simulink model "SC228_TrackedASModelUnitTest"  (R2018b)
settings: Solver=VariableStepAuto  StartTime=0.0  StopTime=10.0  RelTol=1e-3
undefined symbols (not defined in the file or in its folder): ac1dyn_alt0_ft, ac1dyn_con, ac1dyn_lat0_rad, ac1dyn_lon0_rad, ac2dyn_alt0_ft, ac2dyn_con, ac2dyn_lat0_rad, ac2dyn_lon0_rad, ddh_ftps2, dh_ftps, dv_ftps2, e_ft, Edot_ftps, h_ft, hdot_ftps, latLonAltState, n_ft, Ndot_ftps, p_radps, phi_rad, phidot_radps, psi_rad, psidot_radps, q_radps, r_radps, theta_rad, thetadot_radps, uas_tcas_trckd_altQuant_ft, uas_tcas_trckd_bearing_Breakpoints_deg, uas_tcas_trckd_bearing_Max_deg, uas_tcas_trckd_bearing_Sigma_deg, uas_tcas_trckd_dt_s, uas_tcas_trckd_FOR_elev_max_deg, uas_tcas_trckd_FOR_elev_min_deg, uas_tcas_trckd_probDetect, uas_tcas_trckd_psi_bias_ft, uas_tcas_trckd_psi_stddev_ft, uas_tcas_trckd_psidot_bias_radps, uas_tcas_trckd_psidot_stddev_ftps, uas_tcas_trckd_randProbSeed, uas_tcas_trckd_reported_errorCovRBA, uas_tcas_trckd_rng_bias_ft, uas_tcas_trckd_rng_random_stddev_ft, uas_tcas_trckd_seed1, uas_tcas_trckd_seed2, uas_tcas_trckd_seed3, uas_tcas_trckd_seed4, uas_tcas_trckd_sns_max_front_range_ft, uas_tcas_trckd_sns_max_range_ft, uas_tcas_trckd_sns_max_rear_range_ft, uas_tcas_trckd_sns_max_side_range_ft, uas_tcas_trckd_tauThreshold_sec, uas_tcas_trckd_updateRate_sec, v_ftps, vdot_fpss
libraries: simulink x20, dspmtrx3 x1
(part 1 of 2)
settings Model: Creator=PE29732  LastModifiedBy=PE29732

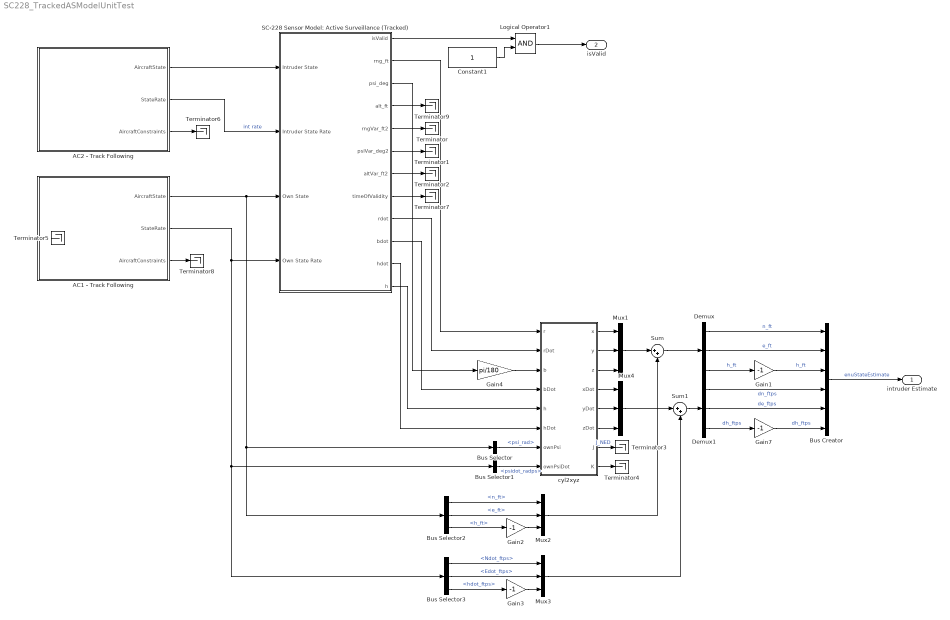
== system SC228_TrackedASModelUnitTest ==
  AC1 - Track Following : Subsystem  mask(Basic Aircraft Dynamic Model){ts_dynamics=0.1, lat0_rad=ac1dyn_lat0_rad, lon0_rad=ac1dyn_lon0_rad, alt_ft=ac1dyn_alt0_ft, v_ftps_max=ac1dyn_con.maxAirspeed_ftps, v_ftps_min=ac1dyn_con.minAirspeed_ftps, dv_ftpss_max=ac1dyn_con.maxAcceleration_ftpss, dv_ftpss_min=ac1dyn_con.minAcceleration_ftpss, dh_ftps_max=ac1dyn_con.maxVerticalRate_ftps, dh_ftps_min=ac1dyn_con.minVerticalRate_ftps, q_radps_max=ac1dyn_con.maxPitchRate_radps, phi_rad_max=ac1dyn_con.maxBankAngle_rad, dphi_radps_max=ac1dyn_con.maxRollRate_radps, r_radps_max=ac1dyn_con.maxYawRate_radps, pNUM=ac1dyn_con.dynamicsNumeratorRollRate, pDEN=ac1dyn_con.dynamicsDenominatorRollRate, hNUM=ac1dyn_con.dynamicsNumeratorVerticalRate, hDEN=ac1dyn_con.dynamicsDenominatorVerticalRate, rNUM=ac1dyn_con.dynamicsNumeratorYawRate, rDEN=ac1dyn_con.dynamicsDenominatorYawRate}
      mask prompts: ts_dynamics "Dynamics update parameter"; lat0_rad "Latitude of ENU origin (rad)"; lon0_rad "Longitude of ENU origin (rad)"; alt_ft "Height of ENU origin (ft)"; v_ftps_max "Maximum airspeed (ft/s)"; v_ftps_min "Minimum airspeed (ft/s)"; dv_ftpss_max "Maximum acceleration (ft/s/s)"; dv_ftpss_min "Miniimum acceleration (ft/s/s)"; dh_ftps_max "Maximum vertical rate (ft/s)"; dh_ftps_min "Minimum vertical rate (ft/s)"; q_radps_max "Maximum pitch rate (rad/s)"; phi_rad_max "Maximum bank angle (rad)"; dphi_radps_max "Maximum roll rate (rad/s)"; r_radps_max "Maximum yaw rate (rad/s)"; pNUM "Roll rate discrete dynamics numerator (2x1)"; pDEN "Roll rate discrete dynamics denominator (1x1)"; hNUM "Vertical rate discrete dynamics numerator (2x1)"; hDEN "Vertical rate discrete dynamics denominator (1x1)"; rNUM "Yaw rate discrete dynamics numerator (2x1)"; rDEN "Yaw rate discrete dynamics denominator (1x1)"
      mask help:
      | Propagates the aircraft dynamics using 6DOF equations of motion.
      |
      | The class Simple6DOF can be used to programmatically set the parameters of Basic Aircraft Dynamcis blocks.
      mask Help:
      | Propagates the aircraft dynamics using 6DOF equations of motion.
      | 
      | The class Simple6DOF can be used to programmatically set the parameters of Basic Aircraft Dynamcis blocks.
      mask DialogControl ParameterTabVar0 Prompt: Main
      mask DialogControl ParameterTabVar01 Prompt: Constraints
  AC2 - Track Following : Subsystem  mask(Basic Aircraft Dynamic Model){ts_dynamics=0.1, lat0_rad=ac2dyn_lat0_rad, lon0_rad=ac2dyn_lon0_rad, alt_ft=ac2dyn_alt0_ft, v_ftps_max=ac2dyn_con.maxAirspeed_ftps, v_ftps_min=ac2dyn_con.minAirspeed_ftps, dv_ftpss_max=ac2dyn_con.maxAcceleration_ftpss, dv_ftpss_min=ac2dyn_con.minAcceleration_ftpss, dh_ftps_max=ac2dyn_con.maxVerticalRate_ftps, dh_ftps_min=ac2dyn_con.minVerticalRate_ftps, q_radps_max=ac2dyn_con.maxPitchRate_radps, phi_rad_max=ac2dyn_con.maxBankAngle_rad, dphi_radps_max=ac2dyn_con.maxRollRate_radps, r_radps_max=ac2dyn_con.maxYawRate_radps, pNUM=ac2dyn_con.dynamicsNumeratorRollRate, pDEN=ac2dyn_con.dynamicsDenominatorRollRate, hNUM=ac2dyn_con.dynamicsNumeratorVerticalRate, hDEN=ac2dyn_con.dynamicsDenominatorVerticalRate, rNUM=ac2dyn_con.dynamicsNumeratorYawRate, rDEN=ac2dyn_con.dynamicsDenominatorYawRate}
      mask prompts: ts_dynamics "Dynamics update parameter"; lat0_rad "Latitude of ENU origin (rad)"; lon0_rad "Longitude of ENU origin (rad)"; alt_ft "Height of ENU origin (ft)"; v_ftps_max "Maximum airspeed (ft/s)"; v_ftps_min "Minimum airspeed (ft/s)"; dv_ftpss_max "Maximum acceleration (ft/s/s)"; dv_ftpss_min "Miniimum acceleration (ft/s/s)"; dh_ftps_max "Maximum vertical rate (ft/s)"; dh_ftps_min "Minimum vertical rate (ft/s)"; q_radps_max "Maximum pitch rate (rad/s)"; phi_rad_max "Maximum bank angle (rad)"; dphi_radps_max "Maximum roll rate (rad/s)"; r_radps_max "Maximum yaw rate (rad/s)"; pNUM "Roll rate discrete dynamics numerator (2x1)"; pDEN "Roll rate discrete dynamics denominator (1x1)"; hNUM "Vertical rate discrete dynamics numerator (2x1)"; hDEN "Vertical rate discrete dynamics denominator (1x1)"; rNUM "Yaw rate discrete dynamics numerator (2x1)"; rDEN "Yaw rate discrete dynamics denominator (1x1)"
      mask help:
      | Propagates the aircraft dynamics using 6DOF equations of motion.
      |
      | The class Simple6DOF can be used to programmatically set the parameters of Basic Aircraft Dynamcis blocks.
      mask Help:
      | Propagates the aircraft dynamics using 6DOF equations of motion.
      | 
      | The class Simple6DOF can be used to programmatically set the parameters of Basic Aircraft Dynamcis blocks.
      mask DialogControl ParameterTabVar0 Prompt: Main
      mask DialogControl ParameterTabVar01 Prompt: Constraints
  Bus Creator : BusCreator  Inputs=6  OutDataTypeStr=Bus: StateEstimate
  Bus Selector : BusSelector  OutputSignals=psi_rad
  Bus Selector1 : BusSelector  OutputSignals=psidot_radps
  Bus Selector2 : BusSelector  OutputSignals=n_ft,e_ft,h_ft
  Bus Selector3 : BusSelector  OutputSignals=Ndot_ftps,Edot_ftps,hdot_ftps
  Constant1 : Constant
  Demux : Demux  Outputs=3
  Demux1 : Demux  Outputs=3
  Gain{1..3,7} (4 alike) : Gain  Gain=-1
  Gain4 : Gain  Gain=pi/180
  Logical Operator1 : Logic  AllPortsSameDT=off  OutDataTypeStr=boolean
  Mux{1..4} (4 alike) : Mux  Inputs=3
  SC-228 Sensor Model: Active Surveillance (Tracked) : Subsystem  mask(Tracked Surveillance: TCAS){dt_s=uas_tcas_trckd_dt_s, lat0_rad=ac1dyn_lat0_rad, lon0_rad=ac1dyn_lon0_rad, alt0_ft=ac1dyn_alt0_ft, sns_max_range_ft=uas_tcas_trckd_sns_max_range_ft, rng_random_stddev_ft=uas_tcas_trckd_rng_random_stddev_ft, rng_bias_ft=uas_tcas_trckd_rng_bias_ft, rng_tau_s=0, seed1=uas_tcas_trckd_seed1, bearing_Max_deg=uas_tcas_trckd_bearing_Max_deg, bearing_Sigma_deg=uas_tcas_trckd_bearing_Sigma_deg, bearing_Breakpoints_deg=uas_tcas_trckd_bearing_Breakpoints_deg, seed2=uas_tcas_trckd_seed2, seed3=uas_tcas_trckd_seed3, seed4=uas_tcas_trckd_seed4, altQuant_ft=uas_tcas_trckd_altQuant_ft, covRBA=uas_tcas_trckd_reported_errorCovRBA, sns_max_front_range_ft=uas_tcas_trckd_sns_max_front_range_ft, sns_max_side_range_ft=uas_tcas_trckd_sns_max_side_range_ft, sns_max_rear_range_ft=uas_tcas_trckd_sns_max_rear_range_ft, probDetect=uas_tcas_trckd_probDetect, FOR_elev_max_deg=uas_tcas_trckd_FOR_elev_max_deg, FOR_elev_min_deg=uas_tcas_trckd_FOR_elev_min_deg, randProbSeed=uas_tcas_trckd_randProbSeed, tauThreshold_sec=uas_tcas_trckd_tauThreshold_sec, updateRate_sec=uas_tcas_trckd_updateRate_sec}
      mask prompts: dt_s "Timestep (s)"; lat0_rad "ENU Reference Latitude (rad)"; lon0_rad "ENU Reference Longitude (rad)"; alt0_ft "ENU Reference Altitude (ft)"; sns_max_range_ft "Sensor Detection Range (ft)"; rng_random_stddev_ft "Random Error Standard Deviation (ft)"; rng_bias_ft "Bias Error (ft)"; rng_tau_s "Correlation Time (s)"; seed1 "Random Seed"; bearing_Max_deg "Bearing Max Error Table (deg)"; bearing_Sigma_deg "Bearing Sigma Table (deg)"; bearing_Breakpoints_deg "Bearing Breakpoints Table (deg)"; seed2 "Random Seed"; seed3 "Lambda Random Seed"; seed4 "Random Seed"; altQuant_ft "Altitude Quantization"; covRBA "Error Covariance Matrix"; sns_max_front_range_ft "Max Detection Range in Front (ft)"; sns_max_side_range_ft "Max Detection Range in Side (ft)"; sns_max_rear_range_ft "Max Detection Range in Back (ft)"; probDetect "Detection Probability"; FOR_elev_max_deg "Max FOR Elevation"; FOR_elev_min_deg "Min FOR Elevation"; randProbSeed "Random Seed"; tauThreshold_sec "Tau Threshold (Change Update Rates) seconds"; updateRate_sec "Update Rate (sec)"
      mask help: Additive noise model of TCAS.
      mask Help:
      | Additive noise model of TCAS. Independent noise is added to each
      | position and velocity component in a range-bearing-altitude coordinate
      | system.  Noise is colored using weights determined by time constant
      | parameters.
      | 
      | Output takes the form of a AircraftEstimate data bus and a 6x6 error covariance
      | matrix in North-East-Down.
      | 
      | Model originally developed for USAF Common ABSAA Program, Nov 2013.
      mask DialogControl ParameterTabVar0 Prompt: Tab
      mask DialogControl ParameterTabVar01 Prompt: Range
      mask DialogControl ParameterTabVar012 Prompt: Bearing
      mask DialogControl ParameterTabVar0123 Prompt: Altitude
      mask DialogControl ParameterTabVar0123456 Prompt: Covariance
      mask DialogControl ParameterTabVar01234567 Prompt: Detection
  Sum : Sum  Inputs=|++
  Sum1 : Sum  Inputs=|++
  Terminator{,1..9} (10 alike) : Terminator
  cyl2xyz : MATLAB Function  TreatAsAtomicUnit=on
  intruder Estimate : Outport
  isValid : Outport  Port=2
  wires:
  SC-228 Sensor Model: Active Surveillance (Tracked)/12(h) -> cyl2xyz/5(h)
  SC-228 Sensor Model: Active Surveillance (Tracked)/1(isValid) -> Logical Operator1/1
  Demux1/2 -> Bus Creator/5  "de_ftps"
  Sum/1 -> Demux/1
  SC-228 Sensor Model: Active Surveillance (Tracked)/9(rdot) -> cyl2xyz/2(rDot)
  Gain4/1 -> cyl2xyz/3(b)
  SC-228 Sensor Model: Active Surveillance (Tracked)/10(bdot) -> cyl2xyz/4(bDot)
  SC-228 Sensor Model: Active Surveillance (Tracked)/5(rngVar_ft2) -> Terminator/1
  Mux4/1 -> Sum1/1
  Bus Selector1/1 -> cyl2xyz/8(ownPsiDot)  "<psidot_radps>"
  cyl2xyz/4(xDot) -> Mux4/1
  cyl2xyz/5(yDot) -> Mux4/2
  Bus Creator/1 -> intruder Estimate/1  "enuStateEstimate"
  Gain1/1 -> Bus Creator/3  "h_ft"
  Gain3/1 -> Mux3/3
  SC-228 Sensor Model: Active Surveillance (Tracked)/6(psiVar_deg2) -> Terminator1/1
  Mux1/1 -> Sum/1
  SC-228 Sensor Model: Active Surveillance (Tracked)/11(hdot) -> cyl2xyz/6(hDot)
  Demux/3 -> Gain1/1  "h_ft"
  Sum1/1 -> Demux1/1
  cyl2xyz/2(y) -> Mux1/2
  SC-228 Sensor Model: Active Surveillance (Tracked)/7(altVar_ft2) -> Terminator2/1
  cyl2xyz/3(z) -> Mux1/3
  Bus Selector/1 -> cyl2xyz/7(ownPsi)  "<psi_rad>"
  SC-228 Sensor Model: Active Surveillance (Tracked)/3(psi_deg) -> Gain4/1
  Mux3/1 -> Sum1/2
  cyl2xyz/8(K) -> Terminator4/1
  Gain7/1 -> Bus Creator/6  "dh_ftps"
  Bus Selector2/2 -> Mux2/2  "<e_ft>"
  cyl2xyz/7(J) -> Terminator3/1  "J_NED"
  Demux1/1 -> Bus Creator/4  "dn_ftps"
  Bus Selector3/2 -> Mux3/2  "<Edot_ftps>"
  AC1 - Track Following/2(StateRate) -> SC-228 Sensor Model: Active Surveillance (Tracked)/4(Own State Rate), Bus Selector1/1, Bus Selector3/1
  cyl2xyz/1(x) -> Mux1/1
  SC-228 Sensor Model: Active Surveillance (Tracked)/2(rng_ft) -> cyl2xyz/1(r)
  Gain2/1 -> Mux2/3
  Mux2/1 -> Sum/2
  Bus Selector2/1 -> Mux2/1  "<n_ft>"
  Demux/2 -> Bus Creator/2  "e_ft"
  cyl2xyz/6(zDot) -> Mux4/3
  Demux1/3 -> Gain7/1  "dh_ftps"
  Demux/1 -> Bus Creator/1  "n_ft"
  Bus Selector3/1 -> Mux3/1  "<Ndot_ftps>"
  Bus Selector2/3 -> Gain2/1  "<h_ft>"
  Logical Operator1/1 -> isValid/1
  Bus Selector3/3 -> Gain3/1  "<hdot_ftps>"
  Constant1/1 -> Logical Operator1/2
  AC1 - Track Following/1(AircraftState) -> SC-228 Sensor Model: Active Surveillance (Tracked)/3(Own State), Bus Selector/1, Bus Selector2/1
  AC2 - Track Following/1(AircraftState) -> SC-228 Sensor Model: Active Surveillance (Tracked)/1(Intruder State)
  AC2 - Track Following/2(StateRate) -> SC-228 Sensor Model: Active Surveillance (Tracked)/2(Intruder State Rate)  "int rate"
  AC2 - Track Following/3(AircraftConstraints) -> Terminator6/1
  SC-228 Sensor Model: Active Surveillance (Tracked)/8(timeOfValidity) -> Terminator7/1
  AC1 - Track Following/3(AircraftConstraints) -> Terminator8/1
  SC-228 Sensor Model: Active Surveillance (Tracked)/4(alt_ft) -> Terminator9/1

== system SC228_TrackedASModelUnitTest/AC1 - Track Following ==
  Follow Trajectory : Subsystem  mask(Follow Trajectory){trajfile=traj1.mat}
      mask prompts: trajfile "Trajectory File Name:"
      mask help: Reads trajectory data (North-East-Altitude position and velocity) from specified file. Computes other state variables to follow that trajectory. Ouptuts AircraftState and AircraftStateRate buses.
      mask init:
      | set_param( [ gcb '/Get Trajectory Data/From File' ], 'Filename', trajfile )
  Performance_constraints : Subsystem
  Rate Transition : RateTransition  OutPortSampleTime=0.1
  AircraftState : Outport  OutDataTypeStr=Bus: AircraftState
  StateRate : Outport  Port=2  OutDataTypeStr=Bus: AircraftStateRate
  AircraftConstraints : Outport  Port=3  OutDataTypeStr=Bus: AircraftConstraints
  wires:
  Follow Trajectory/2(State Rate) -> Rate Transition/1
  Follow Trajectory/1(State) -> AircraftState/1
  Performance_constraints/1(AircraftConstraints) -> Follow Trajectory/1(Constraints), AircraftConstraints/1
  Rate Transition/1 -> StateRate/1

== system SC228_TrackedASModelUnitTest/AC2 - Track Following ==
  Follow Trajectory : Subsystem  mask(Follow Trajectory){trajfile=traj2.mat}
      mask prompts: trajfile "Trajectory File Name:"
      mask help: Reads trajectory data (North-East-Altitude position and velocity) from specified file. Computes other state variables to follow that trajectory. Ouptuts AircraftState and AircraftStateRate buses.
      mask init:
      | set_param( [ gcb '/Get Trajectory Data/From File' ], 'Filename', trajfile )
  Performance_constraints : Subsystem
  Rate Transition : RateTransition  OutPortSampleTime=0.1
  AircraftState : Outport  OutDataTypeStr=Bus: AircraftState
  StateRate : Outport  Port=2  OutDataTypeStr=Bus: AircraftStateRate
  AircraftConstraints : Outport  Port=3  OutDataTypeStr=Bus: AircraftConstraints
  wires:
  Follow Trajectory/2(State Rate) -> Rate Transition/1
  Follow Trajectory/1(State) -> AircraftState/1
  Performance_constraints/1(AircraftConstraints) -> Follow Trajectory/1(Constraints), AircraftConstraints/1
  Rate Transition/1 -> StateRate/1

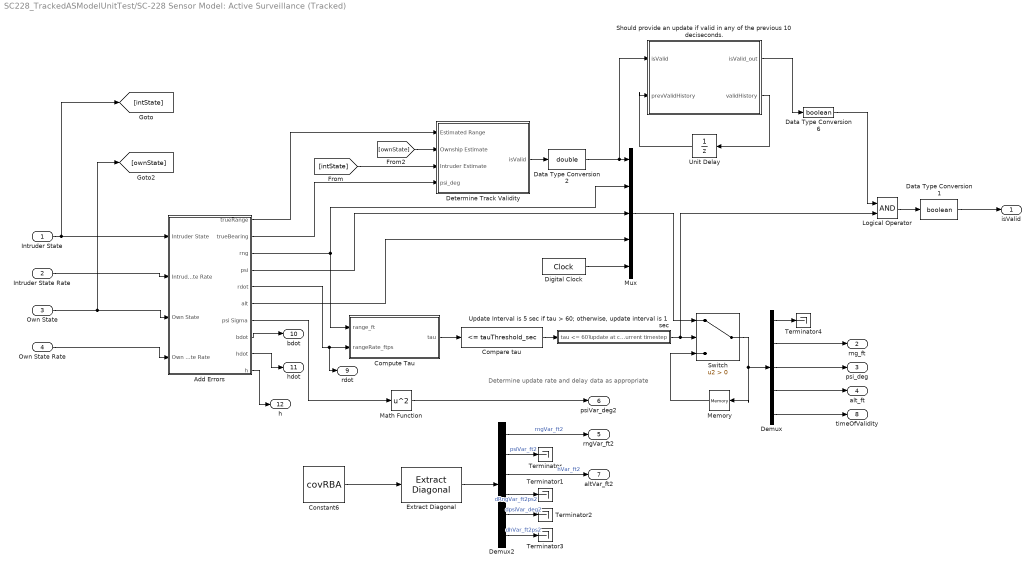
== system SC228_TrackedASModelUnitTest/SC-228 Sensor Model: Active Surveillance (Tracked) ==
  note: Determine update rate and delay data as appropriate
  Intruder State : Inport  OutDataTypeStr=Bus: AircraftState
  Intruder State Rate : Inport  Port=2  OutDataTypeStr=Bus: AircraftStateRate
  Own State : Inport  Port=3  OutDataTypeStr=Bus: AircraftState
  Own State Rate : Inport  Port=4  OutDataTypeStr=Bus: AircraftStateRate
  Add Errors : Subsystem
  Compare tau : simulink/Logic and Bit Operations/Compare To Constant  relop=<=  const=tauThreshold_sec  OutDataTypeStr=boolean
  Compute Tau : Subsystem
  Constant6 : Constant  Value=covRBA
  Data Type Conversion1 : DataTypeConversion  OutDataTypeStr=boolean
  Data Type Conversion2 : DataTypeConversion  OutDataTypeStr=double
  Data Type Conversion6 : DataTypeConversion  OutDataTypeStr=boolean
  Demux : Demux  Outputs=5
  Demux2 : Demux  Outputs=6
  Determine Track Validity : Subsystem
  Digital Clock : DigitalClock  SampleTime=0.1
  Extract Diagonal : dspmtrx3/Extract Diagonal
      settings: SourceProductName=DSP System Toolbox  SourceProductBaseCode=DS
  Logical Operator : Logic  AllPortsSameDT=off  OutDataTypeStr=boolean
  Math Function : Math  Operator=square  SaturateOnIntegerOverflow=on
  Memory : Memory
  Mux : Mux  Inputs=5
  Should provide an update if valid in any of the previous 10 deciseconds. : MATLAB Function  TreatAsAtomicUnit=on
  Switch : Switch  Criteria=u2 > Threshold
  Terminator{,1..4} (5 alike) : Terminator
  Unit Delay : UnitDelay  SampleTime=-1
  "Update Interval is 5 sec if tau > 60; otherwise, update interval is 1 sec" : Subsystem  mask{updateRate=updateRate_sec}
      mask prompts: updateRate "Update Rate When Tau > 60"
  isValid : Outport
  rng_ft : Outport  Port=2
  psi_deg : Outport  Port=3
  alt_ft : Outport  Port=4
  rngVar_ft2 : Outport  Port=5
  psiVar_deg2 : Outport  Port=6
  altVar_ft2 : Outport  Port=7
  timeOfValidity : Outport  Port=8
  rdot : Outport  Port=9
  bdot : Outport  Port=10
  hdot : Outport  Port=11
  h : Outport  Port=12
  wires:
  Add Errors/2(trueBearing) -> Determine Track Validity/4(psi_deg)
  Add Errors/1(trueRange) -> Determine Track Validity/1(Estimated Range)
  Demux/5 -> timeOfValidity/1
  Digital Clock/1 -> Mux/5
  Intruder State/1 -> [intState], Add Errors/1(Intruder State)
  Intruder State Rate/1 -> Add Errors/2(Intruder State Rate)
  Own State/1 -> [ownState], Add Errors/3(Own State)
  Add Errors/3(rng) -> Mux/2, Compute Tau/1(range_ft)
  Own State Rate/1 -> Add Errors/4(Own State Rate)
  [intState] -> Determine Track Validity/3(Intruder Estimate)
  [ownState] -> Determine Track Validity/2(Ownship Estimate)
  Add Errors/6(alt) -> Mux/4
  Add Errors/5(rdot) -> rdot/1, Compute Tau/2(rangeRate_ftps)
  Compute Tau/1(tau) -> Compare tau/1
  Switch/1 -> Memory/1, Demux/1
  Logical Operator/1 -> Data Type Conversion1/1
  Demux/2 -> rng_ft/1
  Demux/3 -> psi_deg/1
  Demux/4 -> alt_ft/1
  Mux/1 -> Switch/1
  Memory/1 -> Switch/3
  Compare tau/1 -> "Update Interval is 5 sec if tau > 60; otherwise, update interval is 1 sec"/1(tau <= 60?)
  Determine Track Validity/1(isValid) -> Data Type Conversion2/1
  Data Type Conversion1/1 -> isValid/1
  Add Errors/7(psi Sigma) -> Math Function/1
  Extract Diagonal/1 -> Demux2/1
  Demux2/4 -> Terminator1/1  "dRngVar_ft2ps2"
  Demux2/5 -> Terminator2/1  "dpsiVar_deg2"
  Demux2/2 -> Terminator/1  "psiVar_ft2"
  Demux2/1 -> rngVar_ft2/1  "rngVar_ft2"
  Constant6/1 -> Extract Diagonal/1
  Demux2/3 -> altVar_ft2/1  "hVar_ft2"
  Demux2/6 -> Terminator3/1  "dhVar_ft2ps2"
  Math Function/1 -> psiVar_deg2/1
  Demux/1 -> Terminator4/1
  "Update Interval is 5 sec if tau > 60; otherwise, update interval is 1 sec"/1(update at current timestep) -> Logical Operator/2, Switch/2
  Should provide an update if valid in any of the previous 10 deciseconds./1(isValid_out) -> Data Type Conversion6/1
  Data Type Conversion2/1 -> Should provide an update if valid in any of the previous 10 deciseconds./1(isValid), Mux/1
  Data Type Conversion6/1 -> Logical Operator/1
  Should provide an update if valid in any of the previous 10 deciseconds./2(validHistory) -> Unit Delay/1
  Unit Delay/1 -> Should provide an update if valid in any of the previous 10 deciseconds./2(prevValidHistory)
  Add Errors/8(bdot) -> bdot/1
  Add Errors/9(hdot) -> hdot/1
  Add Errors/10(h) -> h/1
  Add Errors/4(psi) -> Mux/3

== system SC228_TrackedASModelUnitTest/AC1 - Track Following/Follow Trajectory ==
  Constraints : Inport
  Bus Assignment : BusAssignment  AssignedSignals=p_radps,q_radps,r_radps
  Bus Assignment1 : BusAssignment  AssignedSignals=vdot_fpss,psidot_radps,thetadot_radps,phidot_radps,Ndot_ftps,Edot_ftps,hdot_ftps
  Bus Selector : BusSelector  OutputSignals=dv_ftps2
  Compute Body Rates : Subsystem
  Compute Euler Angles : Subsystem
  Demux : Demux  Outputs=3
  Get Trajectory Data : Subsystem
  Null State Rate : Subsystem
  "Set LLA " : Subsystem  mask{lat0=lat0_rad, lon0=lon0_rad, h0=alt_ft}
      mask prompts: lat0 "ENU latitude origin (rad)"; lon0 "ENU longitude origin (rad)"; h0 "ENU altitude origin (ft)"
  Set State : Subsystem
  Signal Conversion : SignalConversion  OverrideOpt=off
  Signal Conversion1 : SignalConversion  OverrideOpt=off
  State : Outport
  State Rate : Outport  Port=2
  wires:
  Signal Conversion1/1 -> State Rate/1
  Bus Selector/1 -> Bus Assignment1/2  "<dv_ftps2>"
  Compute Euler Angles/3("Phi Dot ") -> Bus Assignment1/5, Compute Body Rates/4(Phi Dot)
  Compute Euler Angles/1(Psi Dot) -> Bus Assignment1/3, Compute Body Rates/2(Psi Dot)
  Demux/3 -> Bus Assignment1/8  "hdot_ftps"
  Null State Rate/1(StateRate) -> Bus Assignment1/1
  Get Trajectory Data/2(xdot) -> Demux/1
  Compute Body Rates/3(r) -> Bus Assignment/4
  Compute Body Rates/2(q) -> Bus Assignment/3
  Compute Body Rates/1(p) -> Bus Assignment/2
  Demux/1 -> Bus Assignment1/6  "Ndot_ftps"
  Demux/2 -> Bus Assignment1/7  "Edot_ftps"
  Compute Euler Angles/2(Theta Dot) -> Bus Assignment1/4, Compute Body Rates/3(Theta Dot)
  Signal Conversion/1 -> State/1
  "Set LLA "/1(State Out) -> Bus Assignment/1
  Bus Assignment/1 -> Signal Conversion/1
  Bus Assignment1/1 -> Signal Conversion1/1
  Set State/1(State) -> Compute Body Rates/1(AircraftState), Compute Euler Angles/1(AircraftState), Bus Selector/1, "Set LLA "/1(State In)
  Constraints/1 -> Compute Euler Angles/2(Constraints)
  Get Trajectory Data/1(x) -> Set State/1(x)

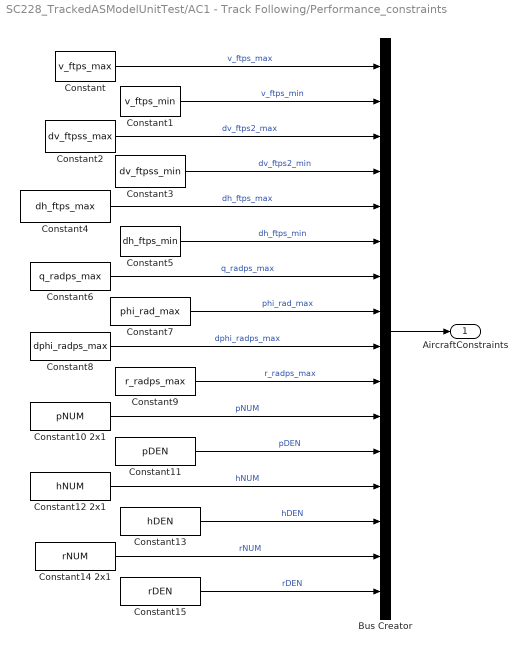
== system SC228_TrackedASModelUnitTest/AC1 - Track Following/Performance_constraints ==
  Bus Creator : BusCreator  Inputs=16
  Constant : Constant  Value=v_ftps_max
  Constant1 : Constant  Value=v_ftps_min
  Constant10 2x1 : Constant  Value=pNUM
  Constant11 : Constant  Value=pDEN
  Constant12 2x1 : Constant  Value=hNUM
  Constant13 : Constant  Value=hDEN
  Constant14 2x1 : Constant  Value=rNUM
  Constant15 : Constant  Value=rDEN
  Constant2 : Constant  Value=dv_ftpss_max
  Constant3 : Constant  Value=dv_ftpss_min
  Constant4 : Constant  Value=dh_ftps_max
  Constant5 : Constant  Value=dh_ftps_min
  Constant6 : Constant  Value=q_radps_max
  Constant7 : Constant  Value=phi_rad_max
  Constant8 : Constant  Value=dphi_radps_max
  Constant9 : Constant  Value=r_radps_max
  AircraftConstraints : Outport  OutDataTypeStr=Bus: AircraftConstraints
  wires:
  Constant10 2x1/1 -> Bus Creator/11  "pNUM"
  Constant12 2x1/1 -> Bus Creator/13  "hNUM"
  Constant14 2x1/1 -> Bus Creator/15  "rNUM"
  Constant8/1 -> Bus Creator/9  "dphi_radps_max"
  Constant7/1 -> Bus Creator/8  "phi_rad_max"
  Constant6/1 -> Bus Creator/7  "q_radps_max"
  Constant5/1 -> Bus Creator/6  "dh_ftps_min"
  Constant4/1 -> Bus Creator/5  "dh_ftps_max"
  Constant3/1 -> Bus Creator/4  "dv_ftps2_min"
  Constant2/1 -> Bus Creator/3  "dv_ftps2_max"
  Constant1/1 -> Bus Creator/2  "v_ftps_min"
  Constant/1 -> Bus Creator/1  "v_ftps_max"
  Bus Creator/1 -> AircraftConstraints/1
  Constant15/1 -> Bus Creator/16  "rDEN"
  Constant13/1 -> Bus Creator/14  "hDEN"
  Constant11/1 -> Bus Creator/12  "pDEN"
  Constant9/1 -> Bus Creator/10  "r_radps_max"

== system SC228_TrackedASModelUnitTest/AC2 - Track Following/Follow Trajectory ==
  Constraints : Inport
  Bus Assignment : BusAssignment  AssignedSignals=p_radps,q_radps,r_radps
  Bus Assignment1 : BusAssignment  AssignedSignals=vdot_fpss,psidot_radps,thetadot_radps,phidot_radps,Ndot_ftps,Edot_ftps,hdot_ftps
  Bus Selector : BusSelector  OutputSignals=dv_ftps2
  Compute Body Rates : Subsystem
  Compute Euler Angles : Subsystem
  Demux : Demux  Outputs=3
  Get Trajectory Data : Subsystem
  Null State Rate : Subsystem
  "Set LLA " : Subsystem  mask{lat0=lat0_rad, lon0=lon0_rad, h0=alt_ft}
      mask prompts: lat0 "ENU latitude origin (rad)"; lon0 "ENU longitude origin (rad)"; h0 "ENU altitude origin (ft)"
  Set State : Subsystem
  Signal Conversion : SignalConversion  OverrideOpt=off
  Signal Conversion1 : SignalConversion  OverrideOpt=off
  State : Outport
  State Rate : Outport  Port=2
  wires:
  Signal Conversion1/1 -> State Rate/1
  Bus Selector/1 -> Bus Assignment1/2  "<dv_ftps2>"
  Compute Euler Angles/3("Phi Dot ") -> Bus Assignment1/5, Compute Body Rates/4(Phi Dot)
  Compute Euler Angles/1(Psi Dot) -> Bus Assignment1/3, Compute Body Rates/2(Psi Dot)
  Demux/3 -> Bus Assignment1/8  "hdot_ftps"
  Null State Rate/1(StateRate) -> Bus Assignment1/1
  Get Trajectory Data/2(xdot) -> Demux/1
  Compute Body Rates/3(r) -> Bus Assignment/4
  Compute Body Rates/2(q) -> Bus Assignment/3
  Compute Body Rates/1(p) -> Bus Assignment/2
  Demux/1 -> Bus Assignment1/6  "Ndot_ftps"
  Demux/2 -> Bus Assignment1/7  "Edot_ftps"
  Compute Euler Angles/2(Theta Dot) -> Bus Assignment1/4, Compute Body Rates/3(Theta Dot)
  Signal Conversion/1 -> State/1
  "Set LLA "/1(State Out) -> Bus Assignment/1
  Bus Assignment/1 -> Signal Conversion/1
  Bus Assignment1/1 -> Signal Conversion1/1
  Set State/1(State) -> Compute Body Rates/1(AircraftState), Compute Euler Angles/1(AircraftState), Bus Selector/1, "Set LLA "/1(State In)
  Constraints/1 -> Compute Euler Angles/2(Constraints)
  Get Trajectory Data/1(x) -> Set State/1(x)

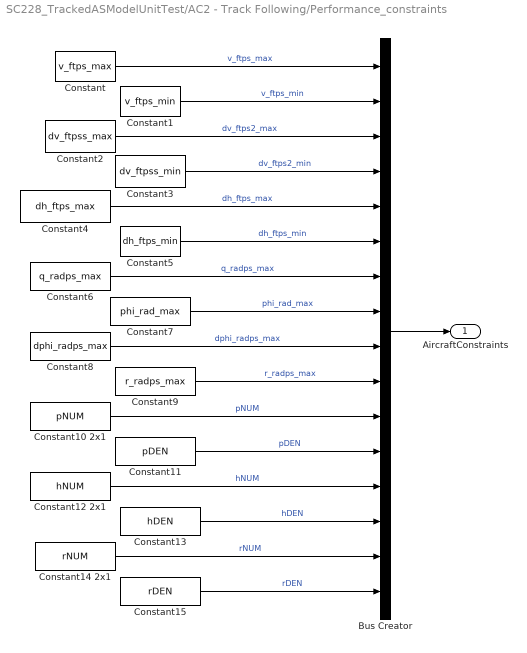
== system SC228_TrackedASModelUnitTest/AC2 - Track Following/Performance_constraints ==
  Bus Creator : BusCreator  Inputs=16
  Constant : Constant  Value=v_ftps_max
  Constant1 : Constant  Value=v_ftps_min
  Constant10 2x1 : Constant  Value=pNUM
  Constant11 : Constant  Value=pDEN
  Constant12 2x1 : Constant  Value=hNUM
  Constant13 : Constant  Value=hDEN
  Constant14 2x1 : Constant  Value=rNUM
  Constant15 : Constant  Value=rDEN
  Constant2 : Constant  Value=dv_ftpss_max
  Constant3 : Constant  Value=dv_ftpss_min
  Constant4 : Constant  Value=dh_ftps_max
  Constant5 : Constant  Value=dh_ftps_min
  Constant6 : Constant  Value=q_radps_max
  Constant7 : Constant  Value=phi_rad_max
  Constant8 : Constant  Value=dphi_radps_max
  Constant9 : Constant  Value=r_radps_max
  AircraftConstraints : Outport  OutDataTypeStr=Bus: AircraftConstraints
  wires:
  Constant10 2x1/1 -> Bus Creator/11  "pNUM"
  Constant12 2x1/1 -> Bus Creator/13  "hNUM"
  Constant14 2x1/1 -> Bus Creator/15  "rNUM"
  Constant8/1 -> Bus Creator/9  "dphi_radps_max"
  Constant7/1 -> Bus Creator/8  "phi_rad_max"
  Constant6/1 -> Bus Creator/7  "q_radps_max"
  Constant5/1 -> Bus Creator/6  "dh_ftps_min"
  Constant4/1 -> Bus Creator/5  "dh_ftps_max"
  Constant3/1 -> Bus Creator/4  "dv_ftps2_min"
  Constant2/1 -> Bus Creator/3  "dv_ftps2_max"
  Constant1/1 -> Bus Creator/2  "v_ftps_min"
  Constant/1 -> Bus Creator/1  "v_ftps_max"
  Bus Creator/1 -> AircraftConstraints/1
  Constant15/1 -> Bus Creator/16  "rDEN"
  Constant13/1 -> Bus Creator/14  "hDEN"
  Constant11/1 -> Bus Creator/12  "pDEN"
  Constant9/1 -> Bus Creator/10  "r_radps_max"

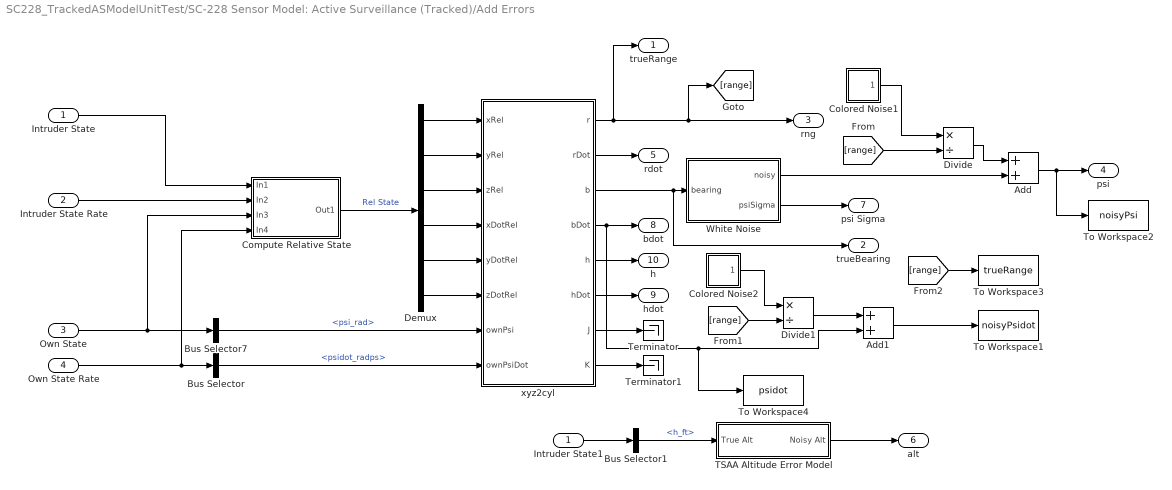
== system SC228_TrackedASModelUnitTest/SC-228 Sensor Model: Active Surveillance (Tracked)/Add Errors ==
  Intruder State : Inport
  Intruder State Rate : Inport  Port=2  OutDataTypeStr=Bus: AircraftStateRate
  Own State : Inport  Port=3
  Own State Rate : Inport  Port=4
  Add : Sum
  Add1 : Sum
  Bus Selector : BusSelector  OutputSignals=psidot_radps
  Bus Selector1 : BusSelector  OutputSignals=h_ft
  Bus Selector7 : BusSelector  OutputSignals=psi_rad
  Colored Noise1 : Subsystem  mask(Colored Noise){sig=uas_tcas_trckd_psi_stddev_ft, bias=uas_tcas_trckd_psi_bias_ft, tau=0, dt=dt_s, seed=seed1}
      mask prompts: sig "Random error standard deviation"; bias "Bias error"; tau "Correlation time"; dt "Track update time"; seed "Random Seed"
      mask help: Generates a noisy state variable estimate using the ABSAA colored noise model. Set correlation time to zero for white noise.
      mask Help:
      | Generates a noisy state variable estimate using the AF Common ABSAA error
      | model.  Time correlation of the error is defined by an exponential decay
      | of K = exp(-tau/dt), where tau is the correlation time and dt is the time
      | between track updates.  The track error at time t is then:
      | 
      |     err(t) = K*err(t-1) + N(0,(1-K^2)*sig^2) + bias
      | 
      | where N(x,y) is a Gaussian noise process with mean x and variance y and
      | with random number generator seeded with the integer 'seed'.
      | 
      | The random noise process must be initialized with an error drawn from
      | N(0,sig^2).
      | 
      | The noise model can be used to produce white noise by setting tau to zero.
  Colored Noise2 : Subsystem  mask(Colored Noise){sig=uas_tcas_trckd_psidot_stddev_ftps, bias=uas_tcas_trckd_psidot_bias_radps, tau=0, dt=dt_s, seed=seed2}
      mask prompts: sig "Random error standard deviation"; bias "Bias error"; tau "Correlation time"; dt "Track update time"; seed "Random Seed"
      mask help: Generates a noisy state variable estimate using the ABSAA colored noise model. Set correlation time to zero for white noise.
      mask Help:
      | Generates a noisy state variable estimate using the AF Common ABSAA error
      | model.  Time correlation of the error is defined by an exponential decay
      | of K = exp(-tau/dt), where tau is the correlation time and dt is the time
      | between track updates.  The track error at time t is then:
      | 
      |     err(t) = K*err(t-1) + N(0,(1-K^2)*sig^2) + bias
      | 
      | where N(x,y) is a Gaussian noise process with mean x and variance y and
      | with random number generator seeded with the integer 'seed'.
      | 
      | The random noise process must be initialized with an error drawn from
      | N(0,sig^2).
      | 
      | The noise model can be used to produce white noise by setting tau to zero.
  Compute Relative State : Subsystem
  Demux : Demux  Outputs=6
  Divide : Product  Inputs=*/
  Divide1 : Product  Inputs=*/
  Intruder State1 : InportShadow
  TSAA Altitude Error Model : Subsystem  AncestorBlock=TSAA_Altitude_Error/TSAA Altitude Error Model  mask{ac_id=1, perfect=false, lambdaSeed=seed3, randomSeed=seed4, altQuant_ft=altQuant_ft, dt_s=0}
      mask prompts: ac_id "Aircraft ID (ownship=1)"; perfect "Use Perfect Altimetry"; lambdaSeed "Lambda Random Seed"; randomSeed "Random Seed"; altQuant_ft "Altitude Quantization (ft)"; dt_s "Sample Time"
  Terminator : Terminator
  Terminator1 : Terminator
  To Workspace1 : ToWorkspace  VariableName=noisyPsidot  SaveFormat=Timeseries  SampleTime=-1
  To Workspace2 : ToWorkspace  VariableName=noisyPsi  SaveFormat=Timeseries  SampleTime=-1
  To Workspace3 : ToWorkspace  VariableName=trueRange  SaveFormat=Timeseries  SampleTime=-1
  To Workspace4 : ToWorkspace  VariableName=psidot  SaveFormat=Timeseries  SampleTime=-1
  White Noise : Subsystem  mask{bearing_Max_deg=bearing_Max_deg, bearing_Sigma_deg=bearing_Sigma_deg, bearing_Breakpoints_deg=bearing_Breakpoints_deg, seed_bearing=seed2}
      mask prompts: bearing_Max_deg "Bearing Max Error Table (deg)"; bearing_Sigma_deg "Bearing Sigma Table (deg)"; bearing_Breakpoints_deg "Bearing Breakpoints Table (deg)"; seed_bearing "Random Seed"
  xyz2cyl : MATLAB Function  TreatAsAtomicUnit=on
  trueRange : Outport
  trueBearing : Outport  Port=2
  rng : Outport  Port=3
  psi : Outport  Port=4
  rdot : Outport  Port=5
  alt : Outport  Port=6
  psi Sigma : Outport  Port=7
  bdot : Outport  Port=8
  hdot : Outport  Port=9
  h : Outport  Port=10
  wires:
  Demux/5 -> xyz2cyl/5(yDotRel)
  Intruder State/1 -> Compute Relative State/1(In1)
  Own State/1 -> Bus Selector7/1, Compute Relative State/3(In3)
  Intruder State Rate/1 -> Compute Relative State/2(In2)
  Bus Selector7/1 -> xyz2cyl/7(ownPsi)  "<psi_rad>"
  Demux/6 -> xyz2cyl/6(zDotRel)
  Compute Relative State/1(Out1) -> Demux/1  "Rel State"
  Demux/1 -> xyz2cyl/1(xRel)
  Demux/3 -> xyz2cyl/3(zRel)
  xyz2cyl/1(r) -> trueRange/1, rng/1, [range]
  xyz2cyl/5(h) -> h/1
  Demux/2 -> xyz2cyl/2(yRel)
  Demux/4 -> xyz2cyl/4(xDotRel)
  Own State Rate/1 -> Compute Relative State/4(In4), Bus Selector/1
  Bus Selector/1 -> xyz2cyl/8(ownPsiDot)  "<psidot_radps>"
  xyz2cyl/7(J) -> Terminator/1
  xyz2cyl/8(K) -> Terminator1/1
  xyz2cyl/2(rDot) -> rdot/1
  xyz2cyl/4(bDot) -> To Workspace4/1, Add1/2, bdot/1
  xyz2cyl/6(hDot) -> hdot/1
  xyz2cyl/3(b) -> trueBearing/1, White Noise/1(bearing)
  White Noise/1("noisy ") -> Add/2
  White Noise/2(psiSigma) -> psi Sigma/1
  Intruder State1/1 -> Bus Selector1/1
  Colored Noise1/1(noisy) -> Divide/1
  Divide/1 -> Add/1
  Add/1 -> To Workspace2/1, psi/1
  Colored Noise2/1(noisy) -> Divide1/1
  Divide1/1 -> Add1/1
  [range] -> Divide/2
  [range] -> Divide1/2
  Add1/1 -> To Workspace1/1
  [range] -> To Workspace3/1
  Bus Selector1/1 -> TSAA Altitude Error Model/1(True Alt)  "<h_ft>"
  TSAA Altitude Error Model/1(Noisy Alt) -> alt/1

== system SC228_TrackedASModelUnitTest/SC-228 Sensor Model: Active Surveillance (Tracked)/Compute Tau ==
  range_ft : Inport
  rangeRate_ftps : Inport  Port=2
  Constant : Constant  Value=9
  Constant1 : Constant  Value=-6
  Divide : Product  Inputs=*/
  Divide1 : Product  Inputs=*/
  Gain : Gain  Gain=1/6070
  Gain1 : Gain  Gain=0.592484
  Gain2 : Gain  Gain=-1
  MinMax : MinMax  Inputs=2
  Subtract : Sum  Inputs=+-
  tau : Outport
  wires:
  rangeRate_ftps/1 -> Gain1/1
  Divide1/1 -> Gain2/1
  range_ft/1 -> Gain/1
  Gain/1 -> Subtract/1, Divide/2
  Constant/1 -> Divide/1
  Divide/1 -> Subtract/2
  Subtract/1 -> Divide1/1
  Gain1/1 -> MinMax/2
  Constant1/1 -> MinMax/1
  MinMax/1 -> Divide1/2
  Gain2/1 -> tau/1

== system SC228_TrackedASModelUnitTest/SC-228 Sensor Model: Active Surveillance (Tracked)/Determine Track Validity ==
  Estimated Range : Inport
  Ownship Estimate : Inport  Port=2
  Intruder Estimate : Inport  Port=3
  psi_deg : Inport  Port=4
  Compute Elevation : Subsystem
  "Determine Validity " : Subsystem  mask{sns_max_front_range_ft=sns_max_front_range_ft, sns_max_side_range_ft=sns_max_side_range_ft, sns_max_rear_range_ft=sns_max_rear_range_ft, FOR_elev_min_deg=FOR_elev_min_deg, FOR_elev_max_deg=FOR_elev_max_deg, probDetect=probDetect}
      mask prompts: sns_max_front_range_ft "Max Front Detection Range (ft)"; sns_max_side_range_ft "Max Side Detection Range (ft)"; sns_max_rear_range_ft "Max Rear Detection Range (ft)"; FOR_elev_min_deg "Min Elevation FOR (deg)"; FOR_elev_max_deg "Max Elevation FOR (deg)"; probDetect "Probability of Detection"
  To Workspace : ToWorkspace  VariableName=elevation_deg  SaveFormat=Timeseries  SampleTime=-1
  Uniform Random Number : UniformRandomNumber  Minimum=0  Seed=randProbSeed  SampleTime=dt_s
  isValid : Outport
  wires:
  Estimated Range/1 -> "Determine Validity "/1(Detection Range)
  Uniform Random Number/1 -> "Determine Validity "/2(Prob Detection)
  "Determine Validity "/1(isValid) -> isValid/1
  Ownship Estimate/1 -> Compute Elevation/1(Ownship Estimate)
  Compute Elevation/1(ElevationOut) -> "Determine Validity "/4(Elevation (deg)), To Workspace/1
  Intruder Estimate/1 -> Compute Elevation/2(Intruder Estimate)
  psi_deg/1 -> "Determine Validity "/3(Bearing (deg))

== system SC228_TrackedASModelUnitTest/SC-228 Sensor Model: Active Surveillance (Tracked)/Update Interval is 5 sec if tau > 60; otherwise, update interval is 1 sec ==
  note: Reset delay
  note: Rate at which block runs out
  tau <= 60? : Inport
  Add1 : Sum
  Constant1 : Constant
  Constant2 : Constant  Value=0
  Delay : Delay  DelayLength=1  InitialCondition=0
  Delay updating if tau > 60 sec : simulink/Logic and Bit Operations/Compare To Constant  relop=>=  const=1/updateRate*1/dt_s  OutDataTypeStr=boolean
  Switch1 : Switch  Criteria=u2 > Threshold
  Switch2 : Switch  Criteria=u2 ~= 0  Threshold=true
  To Workspace : ToWorkspace  VariableName=waitTime  SaveFormat=Timeseries  SampleTime=-1
  To Workspace1 : ToWorkspace  VariableName=TimeToUpdate  SaveFormat=Timeseries  SampleTime=-1
  Unit Delay1 : UnitDelay  InitialCondition=-1  SampleTime=-1
  Update at 1 Hz when tau <= 60 : simulink/Logic and Bit Operations/Compare To Constant  relop=>=  const=1/1*1/dt_s  OutDataTypeStr=boolean
  update at current timestep : Outport
  wires:
  Update at 1 Hz when tau <= 60/1 -> Switch1/1
  Delay updating if tau > 60 sec/1 -> Switch1/3
  tau <= 60?/1 -> Switch1/2
  Delay/1 -> Switch2/2  "Trigger to reset"
  Add1/1 -> Unit Delay1/1, Update at 1 Hz when tau <= 60/1, To Workspace/1, Delay updating if tau > 60 sec/1  "waitTime_s"
  Constant1/1 -> Add1/2
  Unit Delay1/1 -> Switch2/3  "delay_in"
  Constant2/1 -> Switch2/1
  Switch2/1 -> Add1/1  "delay_out"
  Switch1/1 -> update at current timestep/1, Delay/1, To Workspace1/1

== system SC228_TrackedASModelUnitTest/AC1 - Track Following/Follow Trajectory/Compute Body Rates ==
  AircraftState : Inport
  Psi Dot : Inport  Port=2
  Theta Dot : Inport  Port=3
  Phi Dot : Inport  Port=4
  Bus Creator : BusCreator  Inputs=3
  Compute p : Subsystem
  Compute q : Subsystem
  Compute r : Subsystem
  p : Outport
  q : Outport  Port=2
  r : Outport  Port=3
  wires:
  Compute r/1(r) -> r/1
  Compute q/1(q) -> q/1
  Compute p/1(p) -> p/1
  Bus Creator/1 -> Compute p/2(Euler Rates), Compute q/2(Euler Rates), Compute r/2(Euler Rates)
  AircraftState/1 -> Compute p/1(State), Compute q/1(State), Compute r/1(State)
  Psi Dot/1 -> Bus Creator/1  "psidot"
  Phi Dot/1 -> Bus Creator/3  "phidot"
  Theta Dot/1 -> Bus Creator/2  "thetadot"

== system SC228_TrackedASModelUnitTest/AC1 - Track Following/Follow Trajectory/Compute Euler Angles ==
  AircraftState : Inport
  Constraints : Inport  Port=2
  Bus Selector : BusSelector  OutputSignals=psi_rad,theta_rad,phi_rad
  Bus Selector1 : BusSelector  OutputSignals=dphi_radps_max
  Discrete Derivative : simulink/Discrete/Discrete Derivative  gainval=1.0  ICPrevScaledInput=0.0  OutMin=[]  OutMax=[]  OutDataType=fixdt(1, 16)  OutScaling=2^-10  DoSatur=off
  Discrete Derivative1 : simulink/Discrete/Discrete Derivative  gainval=1.0  ICPrevScaledInput=0.0  OutMin=[]  OutMax=[]  OutDataType=fixdt(1, 16)  OutScaling=2^-10  DoSatur=off
  Discrete Derivative2 : simulink/Discrete/Discrete Derivative  gainval=1.0  ICPrevScaledInput=0.0  OutMin=[]  OutMax=[]  OutDataType=fixdt(1, 16)  OutScaling=2^-10  DoSatur=off
  IC : InitialCondition  Value=0
  IC1 : InitialCondition  Value=0
  IC2 : InitialCondition  Value=0
  Saturation Dynamic : simulink/Discontinuities/Saturation Dynamic  OutMin=[]  OutMax=[]  OutDataTypeStr=Inherit: Same as second input  OutDataType=fixdt(1, 16)  OutScaling=2^-10  DoSatur=off
  Unary Minus : UnaryMinus
  Psi Dot : Outport
  Theta Dot : Outport  Port=2
  "Phi Dot " : Outport  Port=3
  wires:
  Constraints/1 -> Bus Selector1/1
  IC2/1 -> Saturation Dynamic/2
  IC1/1 -> Theta Dot/1
  IC/1 -> Psi Dot/1
  Discrete Derivative2/1 -> IC2/1
  Discrete Derivative1/1 -> IC1/1
  Discrete Derivative/1 -> IC/1
  Bus Selector/3 -> Discrete Derivative2/1  "<phi_rad>"
  Bus Selector/2 -> Discrete Derivative1/1  "<theta_rad>"
  Bus Selector/1 -> Discrete Derivative/1  "<psi_rad>"
  AircraftState/1 -> Bus Selector/1
  Saturation Dynamic/1 -> "Phi Dot "/1
  Bus Selector1/1 -> Unary Minus/1, Saturation Dynamic/1  "<dphi_radps_max>"
  Unary Minus/1 -> Saturation Dynamic/3

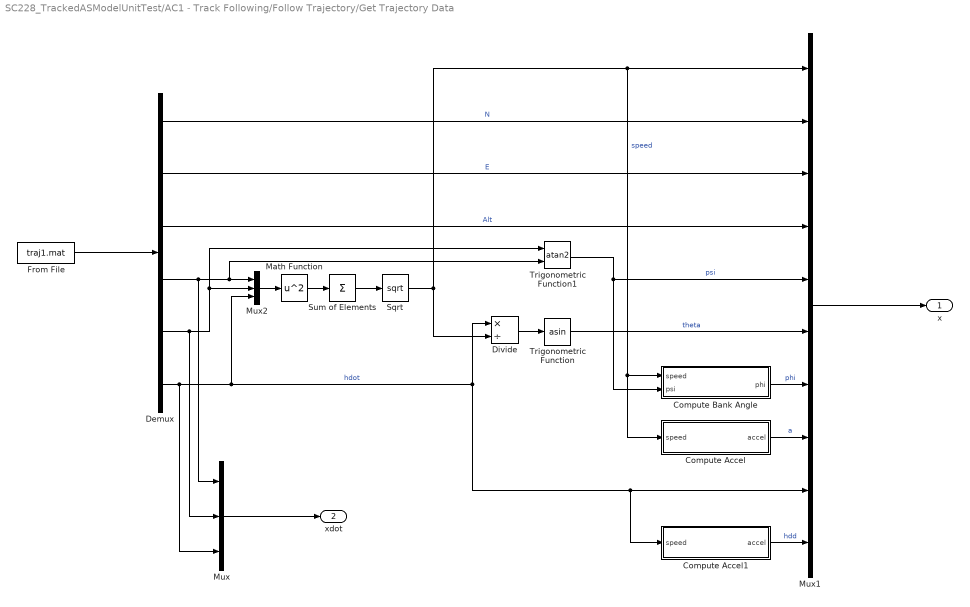
== system SC228_TrackedASModelUnitTest/AC1 - Track Following/Follow Trajectory/Get Trajectory Data ==
  Compute Accel : Subsystem
  Compute Accel1 : Subsystem
  Compute Bank Angle : Subsystem
  Demux : Demux  Outputs=6
  Divide : Product  Inputs=*/
  From File : FromFile  FileName=traj1.mat  SampleTime=0.1
  Math Function : Math  Operator=square  SaturateOnIntegerOverflow=on
  Mux : Mux  Inputs=3
  Mux1 : Mux  Inputs=10
  Mux2 : Mux  Inputs=3
  Sqrt : Sqrt  SaturateOnIntegerOverflow=on
  Sum of Elements : Sum  Inputs=+
  Trigonometric Function : Trigonometry  Operator=asin
  Trigonometric Function1 : Trigonometry  Operator=atan2
  x : Outport
  xdot : Outport  Port=2
  wires:
  Mux/1 -> xdot/1
  Compute Accel1/1(accel) -> Mux1/10  "hdd"
  Demux/5 -> Mux2/2, Trigonometric Function1/1, Mux/2
  Divide/1 -> Trigonometric Function/1
  Trigonometric Function1/1 -> Mux1/5, Compute Bank Angle/2(psi)  "psi"
  Trigonometric Function/1 -> Mux1/6  "theta"
  Compute Bank Angle/1(phi) -> Mux1/7  "phi"
  Compute Accel/1(accel) -> Mux1/8  "a"
  Mux1/1 -> x/1
  Sqrt/1 -> Divide/2, Mux1/1, Compute Bank Angle/1(speed), Compute Accel/1(speed)  "speed"
  Sum of Elements/1 -> Sqrt/1
  Math Function/1 -> Sum of Elements/1
  Mux2/1 -> Math Function/1
  Demux/6 -> Mux1/9, Compute Accel1/1(speed), Divide/1, Mux2/3, Mux/3  "hdot"
  Demux/4 -> Mux2/1, Trigonometric Function1/2, Mux/1
  Demux/3 -> Mux1/4  "Alt"
  Demux/2 -> Mux1/3  "E"
  Demux/1 -> Mux1/2  "N"
  From File/1 -> Demux/1

== system SC228_TrackedASModelUnitTest/AC1 - Track Following/Follow Trajectory/Null State Rate ==
  Bus Creator : BusCreator  Inputs='vdot_fpss','Ndot_ftps','Edot_ftps','hdot_ftps','psidot_radps','thetadot_radps','phidot_radps'  OutDataTypeStr=Bus: AircraftStateRate
  Constant{,1..6} (7 alike) : Constant  Value=0
  StateRate : Outport  OutDataTypeStr=Bus: AircraftStateRate
  wires:
  Constant6/1 -> Bus Creator/7  "phidot_radps"
  Constant5/1 -> Bus Creator/6  "thetadot_radps"
  Constant4/1 -> Bus Creator/5  "psidot_radps"
  Constant3/1 -> Bus Creator/4  "hdot_ftps"
  Constant2/1 -> Bus Creator/3  "Edot_ftps"
  Constant1/1 -> Bus Creator/2  "Ndot_ftps"
  Constant/1 -> Bus Creator/1  "vdot_fpss"
  Bus Creator/1 -> StateRate/1

== system SC228_TrackedASModelUnitTest/AC1 - Track Following/Follow Trajectory/Set LLA  ==
  State In : Inport
  Bus Assignment : BusAssignment  AssignedSignals=latLonAltState.lat_rad,latLonAltState.lon_rad,latLonAltState.dlat_radps,latLonAltState.dlon_radps,latLonAltState.alt_ft,latLonAltState.dalt_ftps
  Bus Selector : BusSelector  OutputSignals=e_ft,n_ft,h_ft,v_ftps,psi_rad,theta_rad
  Constant : Constant  Value=lat0
  Constant7 : Constant  Value=lon0
  Constant8 : Constant  Value=h0
  MATLAB Function : MATLAB Function  TreatAsAtomicUnit=on
  State Out : Outport
  wires:
  Bus Selector/6 -> MATLAB Function/6(theta_rad)  "<theta_rad>"
  Bus Selector/5 -> MATLAB Function/5(psi_rad)  "<psi_rad>"
  Bus Selector/4 -> MATLAB Function/4(v_ftps)  "<v_ftps>"
  Bus Selector/3 -> MATLAB Function/3(u_ft)  "<h_ft>"
  Bus Selector/2 -> MATLAB Function/2(n_ft)  "<n_ft>"
  Bus Selector/1 -> MATLAB Function/1(e_ft)  "<e_ft>"
  Constant8/1 -> MATLAB Function/9(h0)
  Constant7/1 -> MATLAB Function/8(lon0)
  Constant/1 -> MATLAB Function/7(lat0)
  State In/1 -> Bus Selector/1, Bus Assignment/1
  Bus Assignment/1 -> State Out/1
  MATLAB Function/6(dalt_ftps) -> Bus Assignment/7  "dalt_ftps"
  MATLAB Function/5(alt_ft) -> Bus Assignment/6  "alt_ft"
  MATLAB Function/4(dlon_radps) -> Bus Assignment/5  "dlon_radps"
  MATLAB Function/3(dlat_radps) -> Bus Assignment/4  "dlat_radps"
  MATLAB Function/2(lon_rad) -> Bus Assignment/3  "lon_rad"
  MATLAB Function/1(lat_rad) -> Bus Assignment/2  "lat_rad"

== system SC228_TrackedASModelUnitTest/AC1 - Track Following/Follow Trajectory/Set State ==
  x : Inport
  Bus Assignment : BusAssignment  AssignedSignals=v_ftps,n_ft,e_ft,h_ft,psi_rad,theta_rad,phi_rad,dv_ftps2,dh_ftps,ddh_ftps2
  Demux : Demux  Outputs=10
  Null AircraftState : Subsystem
  State : Outport
  wires:
  Demux/10 -> Bus Assignment/11
  Demux/9 -> Bus Assignment/10
  Bus Assignment/1 -> State/1
  Null AircraftState/1(State) -> Bus Assignment/1
  Demux/7 -> Bus Assignment/8  "phi"
  x/1 -> Demux/1
  Demux/6 -> Bus Assignment/7  "theta"
  Demux/5 -> Bus Assignment/6  "psi"
  Demux/4 -> Bus Assignment/5  "h"
  Demux/3 -> Bus Assignment/4  "E"
  Demux/2 -> Bus Assignment/3  "N"
  Demux/1 -> Bus Assignment/2  "v"
  Demux/8 -> Bus Assignment/9  "a"

== system SC228_TrackedASModelUnitTest/AC2 - Track Following/Follow Trajectory/Compute Body Rates ==
  AircraftState : Inport
  Psi Dot : Inport  Port=2
  Theta Dot : Inport  Port=3
  Phi Dot : Inport  Port=4
  Bus Creator : BusCreator  Inputs=3
  Compute p : Subsystem
  Compute q : Subsystem
  Compute r : Subsystem
  p : Outport
  q : Outport  Port=2
  r : Outport  Port=3
  wires:
  Compute r/1(r) -> r/1
  Compute q/1(q) -> q/1
  Compute p/1(p) -> p/1
  Bus Creator/1 -> Compute p/2(Euler Rates), Compute q/2(Euler Rates), Compute r/2(Euler Rates)
  AircraftState/1 -> Compute p/1(State), Compute q/1(State), Compute r/1(State)
  Psi Dot/1 -> Bus Creator/1  "psidot"
  Phi Dot/1 -> Bus Creator/3  "phidot"
  Theta Dot/1 -> Bus Creator/2  "thetadot"

== system SC228_TrackedASModelUnitTest/AC2 - Track Following/Follow Trajectory/Compute Euler Angles ==
  AircraftState : Inport
  Constraints : Inport  Port=2
  Bus Selector : BusSelector  OutputSignals=psi_rad,theta_rad,phi_rad
  Bus Selector1 : BusSelector  OutputSignals=dphi_radps_max
  Discrete Derivative : simulink/Discrete/Discrete Derivative  gainval=1.0  ICPrevScaledInput=0.0  OutMin=[]  OutMax=[]  OutDataType=fixdt(1, 16)  OutScaling=2^-10  DoSatur=off
  Discrete Derivative1 : simulink/Discrete/Discrete Derivative  gainval=1.0  ICPrevScaledInput=0.0  OutMin=[]  OutMax=[]  OutDataType=fixdt(1, 16)  OutScaling=2^-10  DoSatur=off
  Discrete Derivative2 : simulink/Discrete/Discrete Derivative  gainval=1.0  ICPrevScaledInput=0.0  OutMin=[]  OutMax=[]  OutDataType=fixdt(1, 16)  OutScaling=2^-10  DoSatur=off
  IC : InitialCondition  Value=0
  IC1 : InitialCondition  Value=0
  IC2 : InitialCondition  Value=0
  Saturation Dynamic : simulink/Discontinuities/Saturation Dynamic  OutMin=[]  OutMax=[]  OutDataTypeStr=Inherit: Same as second input  OutDataType=fixdt(1, 16)  OutScaling=2^-10  DoSatur=off
  Unary Minus : UnaryMinus
  Psi Dot : Outport
  Theta Dot : Outport  Port=2
  "Phi Dot " : Outport  Port=3
  wires:
  Constraints/1 -> Bus Selector1/1
  IC2/1 -> Saturation Dynamic/2
  IC1/1 -> Theta Dot/1
  IC/1 -> Psi Dot/1
  Discrete Derivative2/1 -> IC2/1
  Discrete Derivative1/1 -> IC1/1
  Discrete Derivative/1 -> IC/1
  Bus Selector/3 -> Discrete Derivative2/1  "<phi_rad>"
  Bus Selector/2 -> Discrete Derivative1/1  "<theta_rad>"
  Bus Selector/1 -> Discrete Derivative/1  "<psi_rad>"
  AircraftState/1 -> Bus Selector/1
  Saturation Dynamic/1 -> "Phi Dot "/1
  Bus Selector1/1 -> Unary Minus/1, Saturation Dynamic/1  "<dphi_radps_max>"
  Unary Minus/1 -> Saturation Dynamic/3

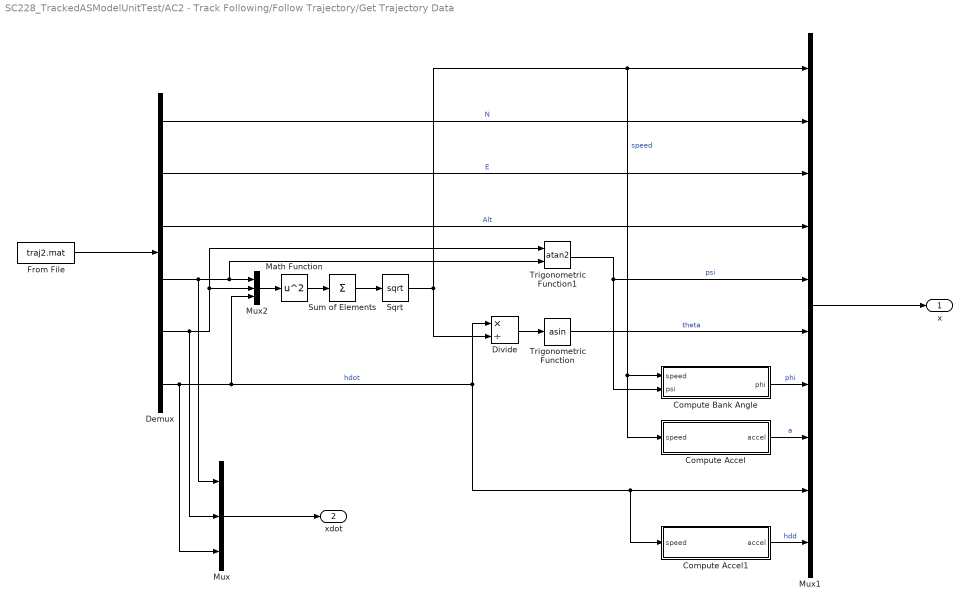
== system SC228_TrackedASModelUnitTest/AC2 - Track Following/Follow Trajectory/Get Trajectory Data ==
  Compute Accel : Subsystem
  Compute Accel1 : Subsystem
  Compute Bank Angle : Subsystem
  Demux : Demux  Outputs=6
  Divide : Product  Inputs=*/
  From File : FromFile  FileName=traj2.mat  SampleTime=0.1
  Math Function : Math  Operator=square  SaturateOnIntegerOverflow=on
  Mux : Mux  Inputs=3
  Mux1 : Mux  Inputs=10
  Mux2 : Mux  Inputs=3
  Sqrt : Sqrt  SaturateOnIntegerOverflow=on
  Sum of Elements : Sum  Inputs=+
  Trigonometric Function : Trigonometry  Operator=asin
  Trigonometric Function1 : Trigonometry  Operator=atan2
  x : Outport
  xdot : Outport  Port=2
  wires:
  Mux/1 -> xdot/1
  Compute Accel1/1(accel) -> Mux1/10  "hdd"
  Demux/5 -> Mux2/2, Trigonometric Function1/1, Mux/2
  Divide/1 -> Trigonometric Function/1
  Trigonometric Function1/1 -> Mux1/5, Compute Bank Angle/2(psi)  "psi"
  Trigonometric Function/1 -> Mux1/6  "theta"
  Compute Bank Angle/1(phi) -> Mux1/7  "phi"
  Compute Accel/1(accel) -> Mux1/8  "a"
  Mux1/1 -> x/1
  Sqrt/1 -> Divide/2, Mux1/1, Compute Bank Angle/1(speed), Compute Accel/1(speed)  "speed"
  Sum of Elements/1 -> Sqrt/1
  Math Function/1 -> Sum of Elements/1
  Mux2/1 -> Math Function/1
  Demux/6 -> Mux1/9, Compute Accel1/1(speed), Divide/1, Mux2/3, Mux/3  "hdot"
  Demux/4 -> Mux2/1, Trigonometric Function1/2, Mux/1
  Demux/3 -> Mux1/4  "Alt"
  Demux/2 -> Mux1/3  "E"
  Demux/1 -> Mux1/2  "N"
  From File/1 -> Demux/1

== system SC228_TrackedASModelUnitTest/AC2 - Track Following/Follow Trajectory/Null State Rate ==
  Bus Creator : BusCreator  Inputs='vdot_fpss','Ndot_ftps','Edot_ftps','hdot_ftps','psidot_radps','thetadot_radps','phidot_radps'  OutDataTypeStr=Bus: AircraftStateRate
  Constant{,1..6} (7 alike) : Constant  Value=0
  StateRate : Outport  OutDataTypeStr=Bus: AircraftStateRate
  wires:
  Constant6/1 -> Bus Creator/7  "phidot_radps"
  Constant5/1 -> Bus Creator/6  "thetadot_radps"
  Constant4/1 -> Bus Creator/5  "psidot_radps"
  Constant3/1 -> Bus Creator/4  "hdot_ftps"
  Constant2/1 -> Bus Creator/3  "Edot_ftps"
  Constant1/1 -> Bus Creator/2  "Ndot_ftps"
  Constant/1 -> Bus Creator/1  "vdot_fpss"
  Bus Creator/1 -> StateRate/1

== system SC228_TrackedASModelUnitTest/AC2 - Track Following/Follow Trajectory/Set LLA  ==
  State In : Inport
  Bus Assignment : BusAssignment  AssignedSignals=latLonAltState.lat_rad,latLonAltState.lon_rad,latLonAltState.dlat_radps,latLonAltState.dlon_radps,latLonAltState.alt_ft,latLonAltState.dalt_ftps
  Bus Selector : BusSelector  OutputSignals=e_ft,n_ft,h_ft,v_ftps,psi_rad,theta_rad
  Constant : Constant  Value=lat0
  Constant7 : Constant  Value=lon0
  Constant8 : Constant  Value=h0
  MATLAB Function : MATLAB Function  TreatAsAtomicUnit=on
  State Out : Outport
  wires:
  Bus Selector/6 -> MATLAB Function/6(theta_rad)  "<theta_rad>"
  Bus Selector/5 -> MATLAB Function/5(psi_rad)  "<psi_rad>"
  Bus Selector/4 -> MATLAB Function/4(v_ftps)  "<v_ftps>"
  Bus Selector/3 -> MATLAB Function/3(u_ft)  "<h_ft>"
  Bus Selector/2 -> MATLAB Function/2(n_ft)  "<n_ft>"
  Bus Selector/1 -> MATLAB Function/1(e_ft)  "<e_ft>"
  Constant8/1 -> MATLAB Function/9(h0)
  Constant7/1 -> MATLAB Function/8(lon0)
  Constant/1 -> MATLAB Function/7(lat0)
  State In/1 -> Bus Selector/1, Bus Assignment/1
  Bus Assignment/1 -> State Out/1
  MATLAB Function/6(dalt_ftps) -> Bus Assignment/7  "dalt_ftps"
  MATLAB Function/5(alt_ft) -> Bus Assignment/6  "alt_ft"
  MATLAB Function/4(dlon_radps) -> Bus Assignment/5  "dlon_radps"
  MATLAB Function/3(dlat_radps) -> Bus Assignment/4  "dlat_radps"
  MATLAB Function/2(lon_rad) -> Bus Assignment/3  "lon_rad"
  MATLAB Function/1(lat_rad) -> Bus Assignment/2  "lat_rad"
